simulink model "hello"  (R2016a)
settings: Solver=ode45  StartTime=0.0  StopTime=100.0  RelTol=1e-3
libraries: fl_lib x10, nesl_utility x5
settings Model: Creator=EDU Student  LastModifiedBy=EDU Student

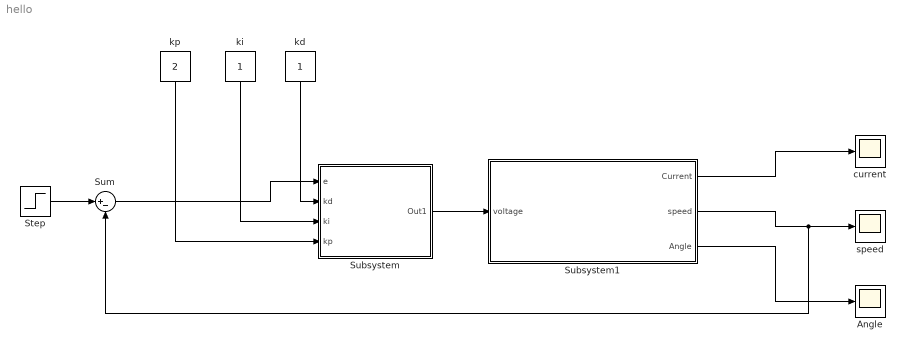
== system hello ==
  Angle : Scope
  Step : Step  SampleTime=0
  Subsystem : Subsystem
  Subsystem1 : Subsystem
  Sum : Sum  Inputs=|+-
  current : Scope
  kd : Constant
  ki : Constant
  kp : Constant  Value=2
  speed : Scope
  wires:
  kp/1 -> Subsystem/4(kp)
  ki/1 -> Subsystem/3(ki)
  kd/1 -> Subsystem/2(kd)
  Subsystem/1(Out1) -> Subsystem1/1(voltage)
  Subsystem1/1(Current) -> current/1
  Subsystem1/2(speed) -> Sum/2, speed/1
  Subsystem1/3(Angle) -> Angle/1
  Step/1 -> Sum/1
  Sum/1 -> Subsystem/1(e)

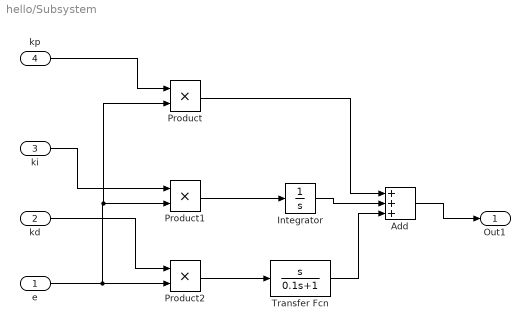
== system hello/Subsystem ==
  e : Inport
  kd : Inport  Port=2
  ki : Inport  Port=3
  kp : Inport  Port=4
  Add : Sum  Inputs=+++
  Integrator : Integrator
  Product : Product
  Product1 : Product
  Product2 : Product
  Transfer Fcn : TransferFcn  Numerator=[1 0]  Denominator=[0.1 1]
  Out1 : Outport
  wires:
  e/1 -> Product/2, Product1/2, Product2/2
  kp/1 -> Product/1
  ki/1 -> Product1/1
  kd/1 -> Product2/1
  Product1/1 -> Integrator/1
  Product/1 -> Add/1
  Integrator/1 -> Add/2
  Product2/1 -> Transfer Fcn/1
  Transfer Fcn/1 -> Add/3
  Add/1 -> Out1/1

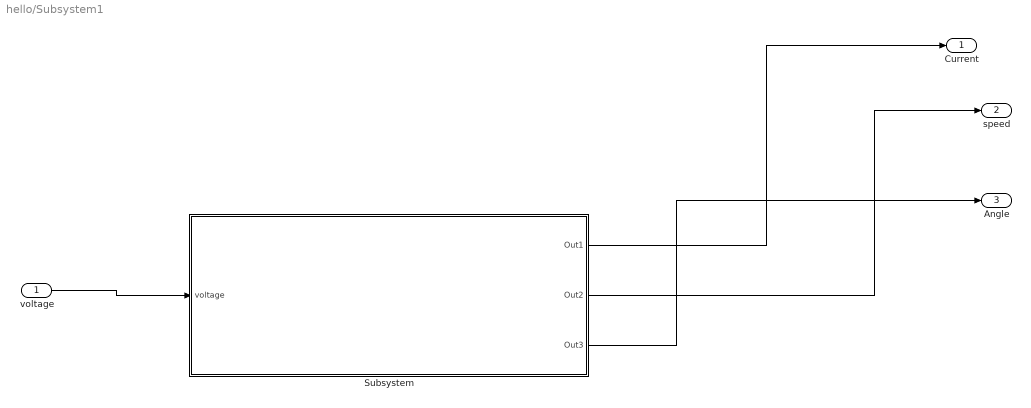
== system hello/Subsystem1 ==
  voltage : Inport
  Subsystem : Subsystem
  Current : Outport
  speed : Outport  Port=2
  Angle : Outport  Port=3
  wires:
  ? -> ?
  voltage/1 -> Subsystem/1(voltage)
  Subsystem/1(Out1) -> Current/1
  Subsystem/2(Out2) -> speed/1
  Subsystem/3(Out3) -> Angle/1

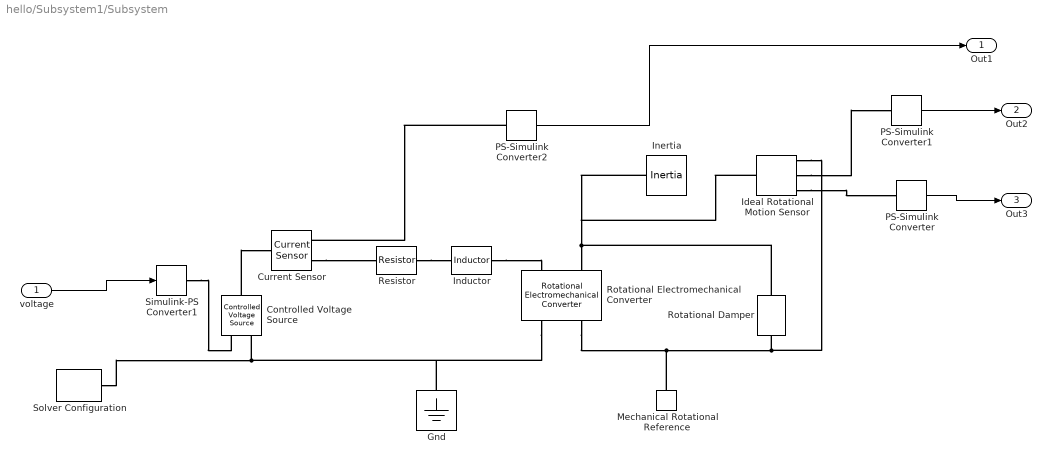
== system hello/Subsystem1/Subsystem ==
  voltage : Inport
  Controlled Voltage Source : fl_lib/Electrical/Electrical Sources/Controlled Voltage Source
  Current Sensor : fl_lib/Electrical/Electrical Sensors/Current Sensor
  Gnd : fl_lib/Electrical/Electrical Elements/Electrical Reference
  Ideal Rotational Motion Sensor : fl_lib/Mechanical/Mechanical Sensors/Ideal Rotational Motion Sensor  offset=0 rad
  Inductor : fl_lib/Electrical/Electrical Elements/Inductor  l=0.5 H  r=0 Ohm  g=1e-9 1/Ohm  i_specify=off  i_priority=None  i=0 A  v_specify=off  v_priority=None  v=0 V  i_L_specify=off  i_L_priority=High  i_L=0 A
  Inertia : fl_lib/Mechanical/Rotational Elements/Inertia  inertia=0.01 kg*m^2  w_specify=off  w_priority=High  w=0 rad/s  t_specify=off  t_priority=None  t=0 N*m
  Mechanical Rotational Reference : fl_lib/Mechanical/Rotational Elements/Mechanical Rotational Reference
  PS-Simulink Converter : nesl_utility/PS-Simulink Converter  PhysicalDomain=network_engine_domain  SubClassName=ps_output  LeftPortType=input  RightPortType=output  PseudoPeriodic=off  Frequencies=[]  Unit=1  AffineConversion=off
  PS-Simulink Converter1 : nesl_utility/PS-Simulink Converter  PhysicalDomain=network_engine_domain  SubClassName=ps_output  LeftPortType=input  RightPortType=output  PseudoPeriodic=off  Frequencies=[]  Unit=1  AffineConversion=off
  PS-Simulink Converter2 : nesl_utility/PS-Simulink Converter  PhysicalDomain=network_engine_domain  SubClassName=ps_output  LeftPortType=input  RightPortType=output  PseudoPeriodic=off  Frequencies=[]  Unit=1  AffineConversion=off
  Resistor : fl_lib/Electrical/Electrical Elements/Resistor  R=1 Ohm  i_specify=off  i_priority=None  i=0 A  v_specify=off  v_priority=None  v=0 V
  Rotational Electromechanical Converter : fl_lib/Electrical/Electrical Elements/Rotational Electromechanical Converter  K=0.01 V/(rad/s)  i_specify=off  i_priority=None  i=0 A  v_specify=off  v_priority=None  v=0 V  t_specify=off  t_priority=None  t=0 N*m  w_specify=off  w_priority=None  w=0 rad/s
  Rotational Damper : fl_lib/Mechanical/Rotational Elements/Rotational Damper  D=0.1 N*m/(rad/s)  w_specify=off  w_priority=None  w=0 rad/s  t_specify=off  t_priority=None  t=0 N*m
  Simulink-PS Converter1 : nesl_utility/Simulink-PS Converter  PhysicalDomain=network_engine_domain  SubClassName=ps_input  LeftPortType=input  RightPortType=output  PseudoPeriodic=off  Frequencies=[]  NoiseDistribution=none  NoiseParameters=[]  Unit=1  AffineConversion=off  InputFiltering=off  SimscapeFilterOrder=1  InputFilterTimeConstant=0.001  UdotUserProvided=1
  Solver Configuration : nesl_utility/Solver Configuration  PhysicalDomain=network_engine_domain  SubClassName=solver  LeftPortType=input  RightPortType=generic  Accelerate=off  Tones=[]  Harmonics=[]  SimulateNoise=off  Profile=off  UseLocalSampling=off  EnableSwitchedLinearOptims=on  FrequencyDomain=off  UseCCode=off  RelTol=0.001  AbsTol=1e-06  MinStep=1e-09  ToWorkspace=off  RevertToSquareIcSolve=off  NumHomotopyIterations=100  PhasorMode=off  PhasorModeNumHarmonics=1  OverrideAbsTol=off  DoDC=off  ResidualTolerance=1e-09  UseLocalSolver=off  LocalSolverChoice=NE_BACKWARD_EULER_ADVANCER  LocalSolverSampleTime=0.001  DoFixedCost=off  MaxNonlinIter=3  MaxModeIter=2  LinearAlgebra=Sparse  DelaysMemoryBudget=1024  AutomaticFiltering=on  FilteringTimeConstant=0.001
  Out1 : Outport
  Out2 : Outport  Port=2
  Out3 : Outport  Port=3
  wires:
  PS-Simulink Converter1/1 -> Out2/1
  PS-Simulink Converter/1 -> Out3/1
  PS-Simulink Converter2/1 -> Out1/1
  voltage/1 -> Simulink-PS Converter1/1
  connections:
  Ideal Rotational Motion Sensor/RConn3 -- PS-Simulink Converter/LConn1
  Solver Configuration/RConn1 -- Gnd/LConn1 -- Rotational Electromechanical Converter/RConn1 -- Controlled Voltage Source/RConn2
  Controlled Voltage Source/LConn1 -- Current Sensor/LConn1
  Ideal Rotational Motion Sensor/RConn2 -- PS-Simulink Converter1/LConn1
  Simulink-PS Converter1/RConn1 -- Controlled Voltage Source/RConn1
  PS-Simulink Converter2/LConn1 -- Current Sensor/RConn1
  Rotational Electromechanical Converter/RConn2 -- Mechanical Rotational Reference/LConn1 -- Ideal Rotational Motion Sensor/RConn1 -- Rotational Damper/RConn1
  Rotational Damper/LConn1 -- Ideal Rotational Motion Sensor/LConn1 -- Inertia/LConn1 -- Rotational Electromechanical Converter/LConn2
  Inductor/RConn1 -- Rotational Electromechanical Converter/LConn1
  Current Sensor/RConn2 -- Resistor/LConn1
  Resistor/RConn1 -- Inductor/LConn1
